simulink model "DTU_Topology_Rural"  (R2023b)
settings: Solver=ode4  StartTime=0.0  StopTime=stoptime  FixedStep=Ts  RelTol=1e-3
PreLoadFcn:
  | Ts=1e-4;load('RuralCase_11052022_12052022_Data_with_ParThreads_Final.mat');run('line_parameters.m');run('Grid_Parameters_3ph.m');
PostLoadFcn:
  | Ts=1e-4;load('RuralCase_11052022_12052022_Data_with_ParThreads_Final.mat');run('line_parameters.m');run('Grid_Parameters_3ph.m');
InitFcn:
  | Ts=1e-4;load('RuralCase_11052022_12052022_Data_with_ParThreads_Final.mat');run('line_parameters.m');run('Grid_Parameters_3ph.m');
StartFcn:
  | Ts=1e-4;load('RuralCase_11052022_12052022_Data_with_ParThreads_Final.mat');run('line_parameters.m');run('Grid_Parameters_3ph.m');
values from neighbouring files (symbols this model uses):
  datastart = 1    [Grid_Parameters_3ph.m]
  datastop = 21556    [Grid_Parameters_3ph.m]
  DTUsignconv = -1000    [Grid_Parameters_3ph.m]
  fnom = 50    [Grid_Parameters_3ph.m]    (also in line_parameters.m)
  line_param = struct()    [line_parameters.m]
  Time = cumsum([0;ones(stoptime,1)])    [Grid_Parameters_3ph.m]
  timestep_meas_data = 1    [Grid_Parameters_3ph.m]
  Vnom = 400    [Grid_Parameters_3ph.m]
undefined symbols (not defined in the file or in its folder): another_event_name, data, j, my_event_name, Newton, Raphson, t_factor
libraries: spsSeriesRLCBranchLib x126, spsGroundLib x71, spsThreePhaseSineGeneratorLib x42, spsControlledCurrentSourceLib x39, spsThreePhaseVIMeasurementLib x26, spsMeanLib x24, spsPowerLib x14, spsMutualInductanceLib x7, rtlab x3, powerlib_meascontrol x3, spsControlledVoltageSourceLib x3, spsThreePhaseSourceLib x1
(part 5 of 5)

== system DTU_Topology_Rural/SM_Master/Uncontrollable Wind Turbine (Gaia)/TrueRMS  ==
  In : Inport
  Mean value : spsMeanLib/Mean  Freq=fnom  Vinit=400^2  Ts=Ts
  Product : Product  InputSameDT=on  SaturateOnIntegerOverflow=on  OutDataTypeStr=Inherit: Same as first input
  Saturation to avoid negative sqrt : Saturate  UpperLimit=Inf  LowerLimit=0
  Sqrt : Sqrt  AlgorithmType=Newton-Raphson
  RMS : Outport  VectorParamsAs1DForOutWhenUnconnected=off
  wires:
  Saturation to avoid negative sqrt/1 -> Sqrt/1
  Mean value/1 -> Saturation to avoid negative sqrt/1
  Product/1 -> Mean value/1
  In/1 -> Product/2, Product/1
  Sqrt/1 -> RMS/1

== system DTU_Topology_Rural/SM_Master/Uncontrollable Wind Turbine (Gaia)/TrueRMS 1 ==
  In : Inport
  Mean value : spsMeanLib/Mean  Freq=fnom  Vinit=0  Ts=Ts
  Product : Product  InputSameDT=on  SaturateOnIntegerOverflow=on  OutDataTypeStr=Inherit: Same as first input
  Saturation to avoid negative sqrt : Saturate  UpperLimit=Inf  LowerLimit=0
  Sqrt : Sqrt  AlgorithmType=Newton-Raphson
  RMS : Outport  VectorParamsAs1DForOutWhenUnconnected=off
  wires:
  Saturation to avoid negative sqrt/1 -> Sqrt/1
  Mean value/1 -> Saturation to avoid negative sqrt/1
  Product/1 -> Mean value/1
  In/1 -> Product/2, Product/1
  Sqrt/1 -> RMS/1
